simulink model "weightlose"  (R2018b)
settings: Solver=VariableStepAuto  StartTime=0.0  StopTime=3000.0  RelTol=1e-3
libraries: cstblocks x1
settings Model: Creator=Administrator  LastModifiedBy=Administrator

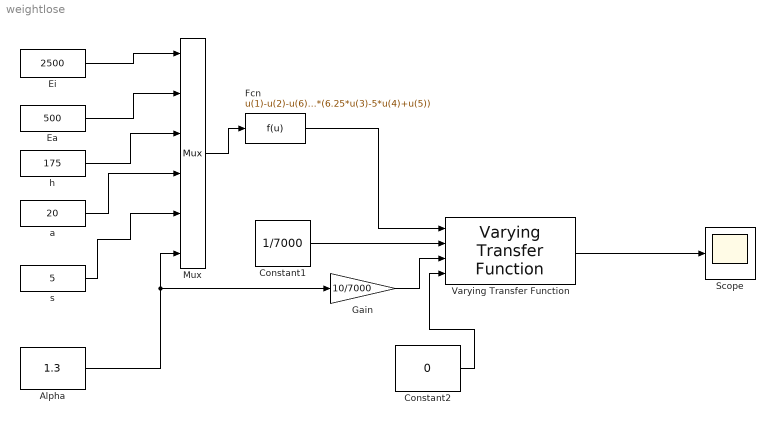
== system weightlose ==
  "Alpha " : Constant  Value=1.3
  Constant1 : Constant  Value=1/7000
  Constant2 : Constant  Value=0
  "Ea " : Constant  Value=500
  "Ei " : Constant  Value=2500
  Fcn : Fcn  Expr=u(1)-u(2)-u(6)*(6.25*u(3)-5*u(4)+u(5))
  Gain : Gain  Gain=10/7000
  Mux : Mux  Inputs=6
  Scope : Scope
  Varying Transfer Function : cstblocks/Linear Parameter Varying/Varying Transfer Function  N=1
      link override Integrator1: InitialCondition=70
      settings: SourceProductName=Control System Toolbox
  a : Constant  Value=20
  h : Constant  Value=175
  "s " : Constant  Value=5
  wires:
  Constant1/1 -> Varying Transfer Function/2
  "Alpha "/1 -> Mux/6, Gain/1
  Gain/1 -> Varying Transfer Function/3
  Constant2/1 -> Varying Transfer Function/4
  "Ei "/1 -> Mux/1
  "Ea "/1 -> Mux/2
  h/1 -> Mux/3
  a/1 -> Mux/4
  "s "/1 -> Mux/5
  Mux/1 -> Fcn/1
  Varying Transfer Function/1 -> Scope/1
  Fcn/1 -> Varying Transfer Function/1
